simulink model "GMCLIB_ElimDcBusRip_BAM_FLT"  (Simulink 8.3)
settings: Solver=ode45  StartTime=0.0  StopTime=10.0  RelTol=1e-3
undefined symbols (not defined in the file): fltModIndex
settings Model: Creator=B17364  LastModifiedBy=B17364
settings DataIOCC: SignalLoggingSaveFormat=Dataset
settings DebuggingCC: UnderspecifiedInitializationDetection=Simplified  StateNameClashWarn=none
settings GRTTargetCC: CombineOutputUpdateFcns=on  GRTInterface=off

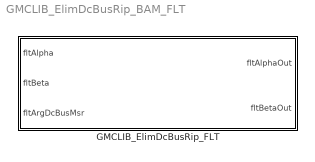
== system GMCLIB_ElimDcBusRip_BAM_FLT ==
  GMCLIB_ElimDcBusRip_FLT : Subsystem  mask(GMCLIB_ElimDcBusRip_FLT){fltModIndex=fltModIndex}
      mask help: Bit accurate model of DC Bus voltage ripple elimination function.
      mask init:
      | pos = get_param(gcb, 'Position');width = pos(3) - pos(1); height = pos(4) - pos(2);tX=width/2;tY=height*0.9;
      mask Display: color('black');port_label('input',1,'fltAlpha');port_label('input',2,'fltBeta');port_label('input',3,'fltArgDcBusMsr');port_label('output',1,'fltAlphaOut');port_label('output',2,'fltBetaOut');color('black');disp('GMCLIB_ElimDcBusRip_FLT');color('blue');text(tX,tY, 'BAM', 'horizontalAlignment', 'center');

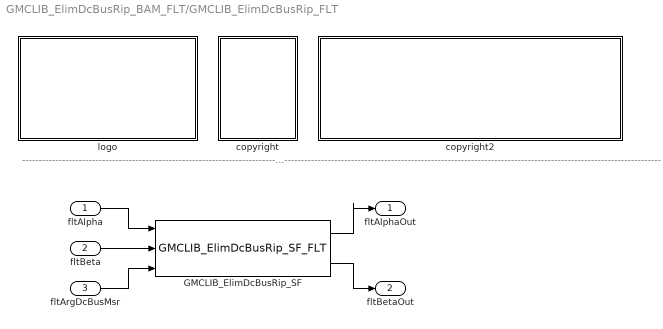
== system GMCLIB_ElimDcBusRip_BAM_FLT/GMCLIB_ElimDcBusRip_FLT ==
  note: ---------------------------------------------------------------------------------------------------------------------------------------------------------------------------------------------------
  fltAlpha : Inport
  fltBeta : Inport  Port=2
  fltArgDcBusMsr : Inport  Port=3
  GMCLIB_ElimDcBusRip_SF : S-Function  FunctionName=GMCLIB_ElimDcBusRip_SF_FLT  Parameters=fltModIndex  EnableBusSupport=off
  copyright : Subsystem
      mask Display: text(10,90,'FILE:');text(10,75,'DESRIPTION:');text(10,60,'COPYRIGHT:');text(10,45,'VERSION:');text(10,30,'DATE:')
  copyright2 : Subsystem
      mask Display: text(10,90,'GMCLIB_ElimDcBusRip_BAM_FLT.mdl');text(10,75,'DC Bus voltage ripple elimination function.');text(10,60,'Freescale');text(10,45,'0.1');text(10,30,'12-Jun-2015');
  logo : Subsystem
      mask Display: image(imread('logo.jpg'))
  fltAlphaOut : Outport
  fltBetaOut : Outport  Port=2
  wires:
  fltAlpha/1 -> GMCLIB_ElimDcBusRip_SF/1
  fltBeta/1 -> GMCLIB_ElimDcBusRip_SF/2
  fltArgDcBusMsr/1 -> GMCLIB_ElimDcBusRip_SF/3
  GMCLIB_ElimDcBusRip_SF/1 -> fltAlphaOut/1
  GMCLIB_ElimDcBusRip_SF/2 -> fltBetaOut/1

== system GMCLIB_ElimDcBusRip_BAM_FLT/GMCLIB_ElimDcBusRip_FLT/copyright ==

== system GMCLIB_ElimDcBusRip_BAM_FLT/GMCLIB_ElimDcBusRip_FLT/copyright2 ==

== system GMCLIB_ElimDcBusRip_BAM_FLT/GMCLIB_ElimDcBusRip_FLT/logo ==
